simulink model "item2"  (R2019a)
settings: Solver=VariableStepAuto  StartTime=0.0  StopTime=30  RelTol=1e-3
libraries: simulink x2
settings Model: Creator=julia  LastModifiedBy=Usuario
settings DataIOCC: ReturnWorkspaceOutputs=off
settings DebuggingCC: ArithmeticOperatorsInVariantConditions=warning
settings SFSimCC: SimUseLocalCustomCode=off
settings RTWCC: RTWUseLocalCustomCode=off
settings CodeAppCC: StateflowObjectComments=on

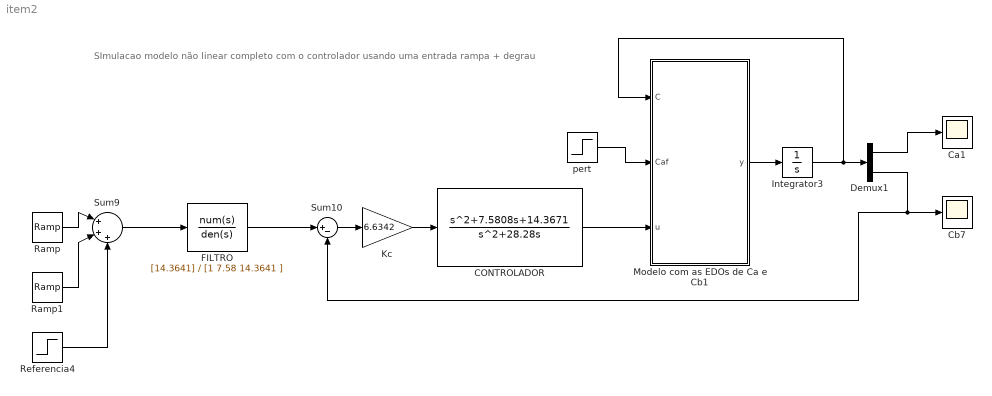
== system item2 ==
  note: SImulacao modelo não linear completo com o controlador
      | usando uma entrada rampa + degrau
  "CONTROLADOR " : TransferFcn  Numerator=[1 7.5808 14.3671]  Denominator=[1 28.28 0]
  Ca1 : Scope
  Cb7 : Scope
  Demux1 : Demux  Outputs=2
  "FILTRO " : TransferFcn  Numerator=[14.3641]  Denominator=[1 7.58 14.3641 ]
  Integrator3 : Integrator  InitialCondition=[0;0]
  "Kc " : Gain  Gain=6.6342
  Modelo com as EDOs de Ca e Cb1 : MATLAB Function  TreatAsAtomicUnit=on
  Ramp : simulink/Sources/Ramp  slope=2.345/5  start=0  InitialOutput=0
  Ramp1 : simulink/Sources/Ramp  slope=-2.345/5  start=5  InitialOutput=0
  Referencia4 : Step  Time=10  After=0.1  SampleTime=0.01
  Sum10 : Sum  Inputs=|+-
  Sum9 : Sum  Inputs=|+++
  "pert    " : Step  Time=20  Before=5.1  After=5.2  SampleTime=0.01
  wires:
  Ramp/1 -> Sum9/1
  Ramp1/1 -> Sum9/2
  Demux1/1 -> Ca1/1
  Demux1/2 -> Sum10/2, Cb7/1
  Modelo com as EDOs de Ca e Cb1/1(y) -> Integrator3/1
  Integrator3/1 -> Modelo com as EDOs de Ca e Cb1/1(C), Demux1/1
  Referencia4/1 -> Sum9/3
  "pert    "/1 -> Modelo com as EDOs de Ca e Cb1/2(Caf)
  Sum10/1 -> "Kc "/1
  "CONTROLADOR "/1 -> Modelo com as EDOs de Ca e Cb1/3(u)
  "Kc "/1 -> "CONTROLADOR "/1
  Sum9/1 -> "FILTRO "/1
  "FILTRO "/1 -> Sum10/1

== matlab function item2/Modelo com as EDOs de Ca e Cb1 ==
  data: y output; C input; Caf input; u input
%EDOs das concentracoes dos produtos A e B
function y = fcn(C, Caf, u)

%constantes
k1 = 6.01; %L/min
k2 = 0.8433; %L/min
k3 = 0.1123; %mol/Lmin

%variaveis das concentracoes dos produtos A e B
Ca = C(1);
Cb = C(2);

%EDOs
Ca_d = -k1*Ca - k3*(Ca^2) + (Caf - Ca)*u;
Cb_d =  k1*Ca - k2*Cb - Cb*u;
 
%conjunto das EDOs
y = [Ca_d;Cb_d];
